simulink model "Partial_shading"  (R2021a)
settings: Solver=VariableStepAuto  StartTime=0.0  StopTime=0.015  RelTol=1e-3
libraries: spsDiodeLib x8, spsPVArrayLib x6, spsGroundLib x2, simulink x2, spsCurrentMeasurementLib x1, spsSeriesRLCBranchLib x1, spsVoltageMeasurementLib x1, spspowerguiLib x1
settings Model: Creator=Anass Soulimani  LastModifiedBy=Anass Soulimani

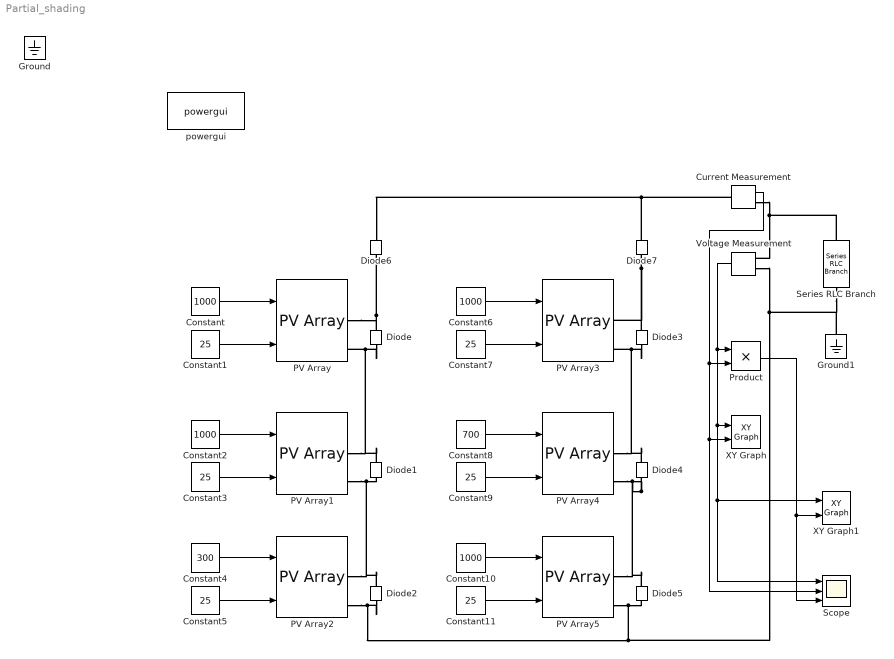
== system Partial_shading ==
  Constant{,2,6,10} (4 alike) : Constant  Value=1000
  Constant{1,3,5,7,9,11} (6 alike) : Constant  Value=25
  Constant4 : Constant  Value=300
  Constant8 : Constant  Value=700
  Current Measurement : spsCurrentMeasurementLib/Current Measurement  PhasorSimulation=off  OutputType=Complex  PSBequivalent=0
  Diode{,1..7} (8 alike) : spsDiodeLib/Diode  Ron=0.001  Lon=0  Vf=0.8  IC=0  UseSnubber=0  Rs=500  Cs=250e-9  Measurements=off
  Ground : spsGroundLib/Ground  LConnTagsString=a
  Ground1 : spsGroundLib/Ground  LConnTagsString=a
  PV Array{,1..5} (6 alike) : spsPVArrayLib/PV Array  Npar=1  Nser=1  PlotType=array @ 1000 W/m2 & specified temperatures  S_vec="[ 1000  500  100 ]"  Temp_C_vec="[ 45 25  ]"  ModuleName=Kyocera Solar KC200GT  PlotWhenSelected=off  Pm=200.143  Ncell=54  Voc=32.9  Isc=8.21  Vm=26.3  Im=7.61  beta_Voc_pc=-0.355  alpha_Isc_pc=0.06  beta_Voc=-0.11679  alpha_Isc=0.004926  IL=8.2288  I0=2.3234e-10  nI=0.97734  Rsh=150.6844  Rs=0.34484  RobustModel=off  RobustCellTemperature=313.3991  BAL=on  Tc=1e-6  Tfilter=5e-5
  Product : Product
  Scope : Scope  NumInputPorts=3
  Series RLC Branch : spsSeriesRLCBranchLib/Series RLC Branch  LConnTagsString=__new0  RConnTagsString=__new0  BranchType=C  Resistance=1  Inductance=1e-3  SetiL0=off  InitialCurrent=0  Capacitance=1e-3  Setx0=off  InitialVoltage=0  Measurements=None
  Voltage Measurement : spsVoltageMeasurementLib/Voltage Measurement  PhasorSimulation=off  OutputType=Complex  PSBequivalent=0
  XY Graph : simulink/Sinks/XY Graph  xmin=0  xmax=100  ymin=0  ymax=18  st=-1
  XY Graph1 : simulink/Sinks/XY Graph  xmin=0  xmax=100  ymin=0  ymax=1300  st=-1
  powergui : spspowerguiLib/powergui  Priority=1  SimulationMode=Continuous  SampleTime=50e-6  frequency=60  Iterations=50  frequencyindice=0  Pbase=100e6  ErrMax=1e-4  UnitsV=kV  UnitsW=MW  buscounter=0  FunctionMessages=off  echomessages=off  EnableUseOfTLC=off  CurrentSourceSwitches=off  DisableSnubberDevices=off  DisableRonSwitches=off  DisableVfSwitches=off  DisplayEquations=off  AutomaticDiscreteSolvers=off  SolverType=Tustin/Backward Euler (TBE)  Interpol=off  ExternalGateDelay=off  methode=off  Ts=100  x0status=blocks  SPID=on  SwTol=0  HookPort=off  NonlinearTolerance=1e-4  nMaxIteration=100  ContinueOnMaxIteration=off  RestoreLinks=warning  ResistiveCurrentMeasurement=off  Frange=[0:2:500]  Ylog=off  Xlog=on  ShowGrid=off  save=off  variable=ZData  structure=0  ZoomFFT=off  StartTime=0.0  cycles=1  DisplayStyle=1  fundamental=60  FreqAxis=off  MaxFrequency=1000  frequencyindicesteady=1  RmsSteady=1  display=off
  wires:
  Constant/1 -> PV Array/1
  Constant1/1 -> PV Array/2
  Constant3/1 -> PV Array1/2
  Constant2/1 -> PV Array1/1
  Constant5/1 -> PV Array2/2
  Constant4/1 -> PV Array2/1
  Constant8/1 -> PV Array4/1
  Constant9/1 -> PV Array4/2
  Constant7/1 -> PV Array3/2
  Constant11/1 -> PV Array5/2
  Constant10/1 -> PV Array5/1
  Constant6/1 -> PV Array3/1
  Current Measurement/1 -> Scope/2, XY Graph/2, Product/2
  Voltage Measurement/1 -> Scope/1, XY Graph1/1, XY Graph/1, Product/1
  Product/1 -> XY Graph1/2, Scope/3
  connections:
  PV Array/RConn1 -- Diode/RConn1 -- Diode6/LConn1
  PV Array1/RConn2 -- Diode2/RConn1 -- PV Array2/RConn1 -- Diode1/LConn1
  Diode/LConn1 -- PV Array1/RConn1 -- Diode1/RConn1 -- PV Array/RConn2
  Diode3/LConn1 -- PV Array3/RConn2 -- PV Array4/RConn1 -- Diode4/RConn1
  Diode4/LConn1 -- Diode5/RConn1 -- PV Array5/RConn1 -- PV Array4/RConn2
  PV Array2/RConn2 -- Ground1/LConn1 -- Series RLC Branch/RConn1 -- Voltage Measurement/LConn2 -- PV Array5/RConn2 -- Diode5/LConn1 -- Diode2/LConn1
  Diode7/LConn1 -- PV Array3/RConn1 -- Diode3/RConn1
  Current Measurement/LConn1 -- Diode7/RConn1 -- Diode6/RConn1
  Current Measurement/RConn1 -- Series RLC Branch/LConn1 -- Voltage Measurement/LConn1
